simulink model "accumulator_thermal_model"  (R2022b)
settings: Solver=VariableStepAuto  StartTime=0.0  StopTime=Tend  RelTol=1e-7  AbsTol=1e-7
InitFcn:
  | HT06_Simulink_Setup
values from neighbouring files (symbols this model uses):
  AH = 18    [HT06_Simulink_Setup.m]
  convectionArea = baseplateArea/126    (= 0.00235277777778)    [Copy_of_Simulink_Setup.m]    (also in HT06_Simulink_Setup.m = 0.00297619047619; Simulink_Setup.m = 0.00297619047619)
  SOC0 = 1    [HT06_Simulink_Setup.m]
  startTempC = 23.5    [Copy_of_Simulink_Setup.m]    (also in HT06_Simulink_Setup.m = 23.3; Simulink_Setup.m)
  tabResis = 0.00009    (= 9e-05)    [Copy_of_Simulink_Setup.m]    (also in HT06_Simulink_Setup.m = 0.0001; Simulink_Setup.m)
undefined symbols (not defined in the file or in its folder): DiscIntNeverNeededParam, S
libraries: fl_lib x49, nesl_utility x18, ee_lib x2
settings Model: Creator=elrii  LastModifiedBy=dknight34
settings SolverCC: AutoScaleAbsTol=off  AlgebraicLoopSolver=TrustRegion
settings DataIOCC: ReturnWorkspaceOutputsName=tp141c3138_a421_409b_bff7_0e00beb78378
settings DebuggingCC: UnconnectedInputMsg=warning  UnconnectedOutputMsg=warning  UnconnectedLineMsg=warning  SymbolicDimsDataTypeCodeGenerationDiagnostic=none  SFMachineParentedDataDiag=warning
settings ModelReferenceCC: EnableRefExpFcnMdlSchedulingChecks=on
settings SFSimCC: CustomCodeUndefinedFunction=UseInterfaceOnly
settings RTWCC: DLArmComputeVersion=19.05
settings SimscapeCC: SimscapeLogType=all  SimscapeLogSimulationStatistics=on  SimscapeLogDataHistory=10000

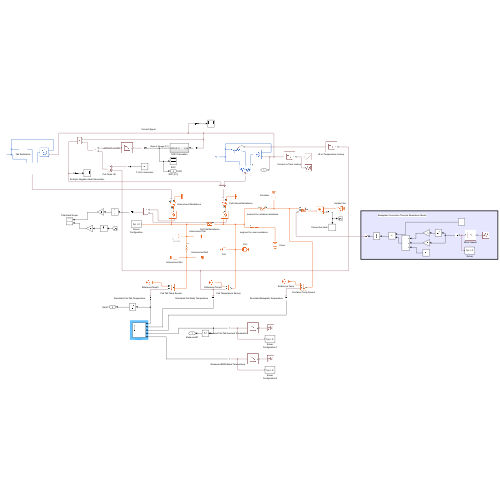
[thumbnail: Simulink's stored preview of the top-level diagram]
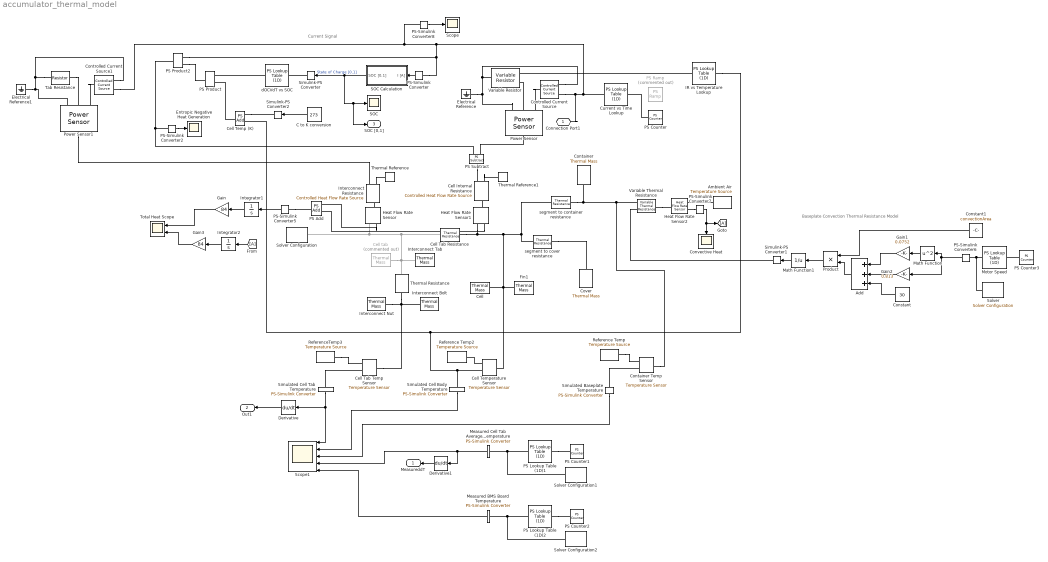
== system accumulator_thermal_model ==
  note: Baseplate Convection Thermal Resistance Model
  note: Current Signal
  " Fin1" : fl_lib/Thermal/Thermal Elements/Thermal Mass  mass=mFin kg  sp_heat=cAl J/kg/K  num_ports=foundation.enum.numPorts2.one  T_specify=on  T_priority=High  T=startTempC degC  T_nominal_specify=off  T_nominal_unit=K  T_nominal_value=1  Q_specify=off  Q_priority=None  Q=0 W  Q_nominal_specify=off  Q_nominal_unit=W  Q_nominal_value=1
  Add : Sum  Inputs=+++
  Ambient Air : fl_lib/Thermal/Thermal Sources/Temperature Source  temperature=startTempC degC
  C to K conversion : Constant  Value=273
  "Cell " : fl_lib/Thermal/Thermal Elements/Thermal Mass  mass=mCell kg  sp_heat=cCell J/kg/K  num_ports=foundation.enum.numPorts2.one  T_specify=on  T_priority=High  T=startTempC degC  T_nominal_specify=off  T_nominal_unit=K  T_nominal_value=1  Q_specify=off  Q_priority=None  Q=0 W  Q_nominal_specify=off  Q_nominal_unit=W  Q_nominal_value=1
  Cell Internal Resistance : fl_lib/Thermal/Thermal Sources/Controlled Heat Flow Rate Source
  Cell Tab Resistance : fl_lib/Thermal/Thermal Elements/Thermal Resistance  resistance=R_tc K/W  T_specify=off  T_priority=None  T=0 K  T_nominal_specify=off  T_nominal_unit=K  T_nominal_value=1  Q_specify=off  Q_priority=None  Q=0 W  Q_nominal_specify=off  Q_nominal_unit=W  Q_nominal_value=1
  Cell Tab Temp Sensor : fl_lib/Thermal/Thermal Sensors/Temperature Sensor
  Cell Temp (K) : fl_lib/Physical Signals/Functions/PS Add
  Cell Temperature Sensor : fl_lib/Thermal/Thermal Sensors/Temperature Sensor
  Cell tab : fl_lib/Thermal/Thermal Elements/Thermal Mass  Commented=on  mass=cellTabThermalMass kg  sp_heat=cCu J/kg/K  num_ports=foundation.enum.numPorts2.one  T_specify=on  T_priority=High  T=startTempC degC  T_nominal_specify=off  T_nominal_unit=K  T_nominal_value=1  Q_specify=off  Q_priority=None  Q=0 W  Q_nominal_specify=off  Q_nominal_unit=W  Q_nominal_value=1
  Constant : Constant  Value=30
  Constant1 : Constant  Value=convectionArea
  Container : fl_lib/Thermal/Thermal Elements/Thermal Mass  mass=mContainerAdj kg  sp_heat=cAl J/kg/K  num_ports=foundation.enum.numPorts2.one  T_specify=on  T_priority=High  T=startTempC degC  T_nominal_specify=off  T_nominal_unit=K  T_nominal_value=1  Q_specify=off  Q_priority=None  Q=0 W  Q_nominal_specify=off  Q_nominal_unit=W  Q_nominal_value=1
  Container Temp Sensor : fl_lib/Thermal/Thermal Sensors/Temperature Sensor
  Controlled Current Source : fl_lib/Electrical/Electrical Sources/Controlled Current Source
  Controlled Current Source1 : fl_lib/Electrical/Electrical Sources/Controlled Current Source
  Convective Heat : Scope
  Cover : fl_lib/Thermal/Thermal Elements/Thermal Mass  mass=mCoverAdj kg  sp_heat=cAl J/kg/K  num_ports=foundation.enum.numPorts2.one  T_specify=on  T_priority=High  T=startTempC degC  T_nominal_specify=off  T_nominal_unit=K  T_nominal_value=1  Q_specify=off  Q_priority=None  Q=0 W  Q_nominal_specify=off  Q_nominal_unit=W  Q_nominal_value=1
  Current vs Time Lookup : fl_lib/Physical Signals/Lookup Tables/PS Lookup Table (1D)  x=emTime  f=emCurrent A  interp_method=simscape.enum.interpolation.linear  extrap_method=simscape.enum.extrapolation.nearest
  Derivative : Derivative
  Derivative1 : Derivative
  Electrical Reference : fl_lib/Electrical/Electrical Elements/Electrical Reference
  Electrical Reference1 : fl_lib/Electrical/Electrical Elements/Electrical Reference
  Entropic Negative Heat Generation : Scope
  From : From
  Gain : Gain  Gain=84
  Gain1 : Gain  Gain=0.0752
  Gain2 : Gain  Gain=0.813
  Gain3 : Gain  Gain=84
  Goto : Goto
  Heat Flow Rate Sensor : fl_lib/Thermal/Thermal Sensors/Heat Flow Rate Sensor
  Heat Flow Rate Sensor1 : fl_lib/Thermal/Thermal Sensors/Heat Flow Rate Sensor
  Heat Flow Rate Sensor2 : fl_lib/Thermal/Thermal Sensors/Heat Flow Rate Sensor
  IR vs Temperature Lookup : fl_lib/Physical Signals/Lookup Tables/PS Lookup Table (1D)  x=tempVec K  f=IRVec Ohm  interp_method=simscape.enum.interpolation.linear  extrap_method=simscape.enum.extrapolation.nearest
  Integrator1 : Integrator
  Integrator2 : Integrator
  Interconnect Bolt : fl_lib/Thermal/Thermal Elements/Thermal Mass  mass=mInterconnectBoltTotal kg  sp_heat=cSt J/kg/K  num_ports=foundation.enum.numPorts2.one  T_specify=on  T_priority=High  T=startTempC degC  T_nominal_specify=off  T_nominal_unit=K  T_nominal_value=1  Q_specify=off  Q_priority=None  Q=0 W  Q_nominal_specify=off  Q_nominal_unit=W  Q_nominal_value=1
  Interconnect Nut : fl_lib/Thermal/Thermal Elements/Thermal Mass  mass=mInterconnectNutTotal kg  sp_heat=cSt J/kg/K  num_ports=foundation.enum.numPorts2.one  T_specify=on  T_priority=High  T=startTempC degC  T_nominal_specify=off  T_nominal_unit=K  T_nominal_value=1  Q_specify=off  Q_priority=None  Q=0 W  Q_nominal_specify=off  Q_nominal_unit=W  Q_nominal_value=1
  Interconnect Resistance : fl_lib/Thermal/Thermal Sources/Controlled Heat Flow Rate Source
  Interconnect Tab : fl_lib/Thermal/Thermal Elements/Thermal Mass  mass=mInterconnect kg  sp_heat=cAl J/kg/K  num_ports=foundation.enum.numPorts2.one  T_specify=on  T_priority=High  T=startTempC degC  T_nominal_specify=off  T_nominal_unit=K  T_nominal_value=1  Q_specify=off  Q_priority=None  Q=0 W  Q_nominal_specify=off  Q_nominal_unit=W  Q_nominal_value=1
  Math Function : Math  Operator=square
  Math Function1 : Math  Operator=reciprocal
  Measured BMS Board Temperature : nesl_utility/PS-Simulink Converter  PhysicalDomain=network_engine_domain  SubClassName=ps_output  LeftPortType=input  RightPortType=output  PseudoPeriodic=off  Frequencies=[]  VectorFormat=1-D array  Unit=inherit  AffineConversion=off
  Measured Cell Tab Average Temperature : nesl_utility/PS-Simulink Converter  PhysicalDomain=network_engine_domain  SubClassName=ps_output  LeftPortType=input  RightPortType=output  PseudoPeriodic=off  Frequencies=[]  VectorFormat=1-D array  Unit=inherit  AffineConversion=off
  Motor Speed : fl_lib/Physical Signals/Lookup Tables/PS Lookup Table (1D)  x=S.vehicle_speed(:,1)  f=S.vehicle_speed(:,2)  interp_method=simscape.enum.interpolation.linear  extrap_method=simscape.enum.extrapolation.nearest
  PS Add : fl_lib/Physical Signals/Functions/PS Add
  PS Counter : fl_lib/Physical Signals/Sources/PS Counter  sample_time=1 s  init_val=0  reset_val=0  max_val=intmax
      settings: InternalSimscapePortConfiguration="{\"Bottom\":[],\"Left\":[],\"Right\":[{\"id\":\"Y\",\"label\":\"Y\",\"type\":\"output\"}],\"Top\":[]}"
  PS Counter1 : fl_lib/Physical Signals/Sources/PS Counter  sample_time=1 s  init_val=1  reset_val=0  max_val=100000
      settings: InternalSimscapePortConfiguration="{\"Bottom\":[],\"Left\":[],\"Right\":[{\"id\":\"Y\",\"label\":\"Y\",\"type\":\"output\"}],\"Top\":[]}"
  PS Counter2 : fl_lib/Physical Signals/Sources/PS Counter  sample_time=1 s  init_val=1  reset_val=0  max_val=100000
      settings: InternalSimscapePortConfiguration="{\"Bottom\":[],\"Left\":[],\"Right\":[{\"id\":\"Y\",\"label\":\"Y\",\"type\":\"output\"}],\"Top\":[]}"
  PS Counter3 : fl_lib/Physical Signals/Sources/PS Counter  sample_time=1 s  init_val=0  reset_val=0  max_val=intmax
      settings: InternalSimscapePortConfiguration="{\"Bottom\":[],\"Left\":[],\"Right\":[{\"id\":\"Y\",\"label\":\"Y\",\"type\":\"output\"}],\"Top\":[]}"
  PS Lookup Table (1D)1 : fl_lib/Physical Signals/Lookup Tables/PS Lookup Table (1D)  x=time  f=tempInterp  interp_method=simscape.enum.interpolation.linear  extrap_method=simscape.enum.extrapolation.nearest
  PS Lookup Table (1D)2 : fl_lib/Physical Signals/Lookup Tables/PS Lookup Table (1D)  x=time  f=accAirTempInterp  interp_method=simscape.enum.interpolation.linear  extrap_method=simscape.enum.extrapolation.nearest
  PS Product : fl_lib/Physical Signals/Functions/PS Product
  PS Product2 : fl_lib/Physical Signals/Functions/PS Product
  PS Ramp : fl_lib/Physical Signals/Sources/PS Ramp  Commented=on  slope=1 1/s  start_time=0 s  initial_output=0
  PS Subtract : fl_lib/Physical Signals/Functions/PS Subtract
  PS-Simulink Converter : nesl_utility/PS-Simulink Converter  PhysicalDomain=network_engine_domain  SubClassName=ps_output  LeftPortType=input  RightPortType=output  PseudoPeriodic=off  Frequencies=[]  VectorFormat=1-D array  Unit=inherit  AffineConversion=off
  PS-Simulink Converter2 : nesl_utility/PS-Simulink Converter  PhysicalDomain=network_engine_domain  SubClassName=ps_output  LeftPortType=input  RightPortType=output  PseudoPeriodic=off  Frequencies=[]  VectorFormat=1-D array  Unit=inherit  AffineConversion=off
  PS-Simulink Converter5 : nesl_utility/PS-Simulink Converter  PhysicalDomain=network_engine_domain  SubClassName=ps_output  LeftPortType=input  RightPortType=output  PseudoPeriodic=off  Frequencies=[]  VectorFormat=1-D array  Unit=inherit  AffineConversion=off
  PS-Simulink Converter6 : nesl_utility/PS-Simulink Converter  PhysicalDomain=network_engine_domain  SubClassName=ps_output  LeftPortType=input  RightPortType=output  PseudoPeriodic=off  Frequencies=[]  VectorFormat=inherit  Unit=inherit  AffineConversion=off
  PS-Simulink Converter7 : nesl_utility/PS-Simulink Converter  PhysicalDomain=network_engine_domain  SubClassName=ps_output  LeftPortType=input  RightPortType=output  PseudoPeriodic=off  Frequencies=[]  VectorFormat=inherit  Unit=inherit  AffineConversion=off
  PS-Simulink Converter8 : nesl_utility/PS-Simulink Converter  PhysicalDomain=network_engine_domain  SubClassName=ps_output  LeftPortType=input  RightPortType=output  PseudoPeriodic=off  Frequencies=[]  VectorFormat=inherit  Unit=inherit  AffineConversion=off
  Power Sensor : ee_lib/Sensors & Transducers/Power Sensor  measurement_type=1  averaging_period=1e-4 s
  Power Sensor1 : ee_lib/Sensors & Transducers/Power Sensor  measurement_type=1  averaging_period=1e-4 s
  Product : Product
  Reference Temp : fl_lib/Thermal/Thermal Sources/Temperature Source  temperature=0 degC
  Reference Temp2 : fl_lib/Thermal/Thermal Sources/Temperature Source  temperature=0 degC
  ReferenceTemp3 : fl_lib/Thermal/Thermal Sources/Temperature Source  temperature=0 degC
  SOC : Scope
  SOC Calculation : Subsystem
  Scope : Scope
  Scope1 : Scope  NumInputPorts=5
  Simulated Baseplate Temperature : nesl_utility/PS-Simulink Converter  PhysicalDomain=network_engine_domain  SubClassName=ps_output  LeftPortType=input  RightPortType=output  PseudoPeriodic=off  Frequencies=[]  VectorFormat=1-D array  Unit=inherit  AffineConversion=off
  Simulated Cell Body Temperature : nesl_utility/PS-Simulink Converter  PhysicalDomain=network_engine_domain  SubClassName=ps_output  LeftPortType=input  RightPortType=output  PseudoPeriodic=off  Frequencies=[]  VectorFormat=1-D array  Unit=inherit  AffineConversion=off
  Simulated Cell Tab Temperature : nesl_utility/PS-Simulink Converter  PhysicalDomain=network_engine_domain  SubClassName=ps_output  LeftPortType=input  RightPortType=output  PseudoPeriodic=off  Frequencies=[]  VectorFormat=1-D array  Unit=inherit  AffineConversion=off
  Simulink-PS Converter : nesl_utility/Simulink-PS Converter  PhysicalDomain=network_engine_domain  SubClassName=ps_input  LeftPortType=input  RightPortType=output  PseudoPeriodic=off  Frequencies=[]  NoiseDistribution=none  NoiseParameters=[]  Unit=1  AffineConversion=off  FilteringAndDerivatives=provide  SimscapeFilterOrder=1  InputFilterTimeConstant=0.001  UdotUserProvided=0
  Simulink-PS Converter1 : nesl_utility/Simulink-PS Converter  PhysicalDomain=network_engine_domain  SubClassName=ps_input  LeftPortType=input  RightPortType=output  PseudoPeriodic=off  Frequencies=[]  NoiseDistribution=none  NoiseParameters=[]  Unit=K/W  AffineConversion=off  FilteringAndDerivatives=provide  SimscapeFilterOrder=1  InputFilterTimeConstant=0.001  UdotUserProvided=0
  Simulink-PS Converter2 : nesl_utility/Simulink-PS Converter  PhysicalDomain=network_engine_domain  SubClassName=ps_input  LeftPortType=input  RightPortType=output  PseudoPeriodic=off  Frequencies=[]  NoiseDistribution=none  NoiseParameters=[]  Unit=K  AffineConversion=off  FilteringAndDerivatives=provide  SimscapeFilterOrder=1  InputFilterTimeConstant=0.001  UdotUserProvided=0
  Solver : nesl_utility/Solver Configuration  PhysicalDomain=network_engine_domain  SubClassName=solver  LeftPortType=input  RightPortType=generic  Tones=[]  Harmonics=[]  SimulateNoise=off  Profile=off  UseLocalSampling=off  EnableSwitchedLinearOptims=on  FrequencyDomain=off  UseCCode=off  RelTol=0.001  AbsTol=1e-06  MinStep=1e-09  ToWorkspace=off  RevertToSquareIcSolve=off  NumHomotopyIterations=100  PhasorMode=off  PhasorModeNumHarmonics=1  ConsistencySolver=NEWTON_FTOL  IndexReductionMethod=DerivativeReplacement  DoDC=off  ResidualTolerance=1e-09  ConsistencyTolSource=GLOBAL  ConsistencyAbsTol=0.001  ConsistencyRelTol=0.001  ConsistencyTolFactor=0.001  UseLocalSolver=off  LocalSolverChoice=NE_BACKWARD_EULER_ADVANCER  ResolveIndetEquations=on  FunctionEvalNumThread=1  LocalSolverSampleTime=0.001  DoFixedCost=off  MaxNonlinIter=3  MaxModeIter=2  ComputeImpulses=off  ImpulseIterations=2  LinearAlgebra=auto  LinearAlgebraNumThread=0  EquationFormulation=NE_TIME_EF  DelaysMemoryBudget=1024  AutomaticFiltering=on  FilteringTimeConstant=0.001  PartitionStorageMethod=AS_NEEDED  PartitionMemoryBudget=1024  PartitionMethod=ROBUST
  Solver Configuration : nesl_utility/Solver Configuration  PhysicalDomain=network_engine_domain  SubClassName=solver  LeftPortType=input  RightPortType=generic  Tones=[]  Harmonics=[]  SimulateNoise=off  Profile=off  UseLocalSampling=off  EnableSwitchedLinearOptims=on  FrequencyDomain=off  UseCCode=off  RelTol=0.001  AbsTol=1e-06  MinStep=1e-09  ToWorkspace=off  RevertToSquareIcSolve=off  NumHomotopyIterations=100  PhasorMode=off  PhasorModeNumHarmonics=1  ConsistencySolver=NEWTON_FTOL  IndexReductionMethod=DerivativeReplacement  DoDC=off  ResidualTolerance=1e-012  ConsistencyTolSource=GLOBAL  ConsistencyAbsTol=0.001  ConsistencyRelTol=0.001  ConsistencyTolFactor=0.001  UseLocalSolver=off  LocalSolverChoice=NE_BACKWARD_EULER_ADVANCER  ResolveIndetEquations=on  FunctionEvalNumThread=1  LocalSolverSampleTime=0.001  DoFixedCost=off  MaxNonlinIter=3  MaxModeIter=2  ComputeImpulses=off  ImpulseIterations=2  LinearAlgebra=auto  LinearAlgebraNumThread=0  EquationFormulation=NE_TIME_EF  DelaysMemoryBudget=1024  AutomaticFiltering=on  FilteringTimeConstant=0.001  PartitionStorageMethod=AS_NEEDED  PartitionMemoryBudget=1024  PartitionMethod=ROBUST
  Solver Configuration1 : nesl_utility/Solver Configuration  PhysicalDomain=network_engine_domain  SubClassName=solver  LeftPortType=input  RightPortType=generic  Tones=[]  Harmonics=[]  SimulateNoise=off  Profile=off  UseLocalSampling=off  EnableSwitchedLinearOptims=on  FrequencyDomain=off  UseCCode=off  RelTol=0.001  AbsTol=1e-06  MinStep=1e-09  ToWorkspace=off  RevertToSquareIcSolve=off  NumHomotopyIterations=100  PhasorMode=off  PhasorModeNumHarmonics=1  ConsistencySolver=NEWTON_FTOL  IndexReductionMethod=DerivativeReplacement  DoDC=off  ResidualTolerance=1e-09  ConsistencyTolSource=GLOBAL  ConsistencyAbsTol=0.001  ConsistencyRelTol=0.001  ConsistencyTolFactor=0.001  UseLocalSolver=off  LocalSolverChoice=NE_BACKWARD_EULER_ADVANCER  ResolveIndetEquations=on  FunctionEvalNumThread=1  LocalSolverSampleTime=0.001  DoFixedCost=off  MaxNonlinIter=3  MaxModeIter=2  ComputeImpulses=off  ImpulseIterations=2  LinearAlgebra=auto  LinearAlgebraNumThread=0  EquationFormulation=NE_TIME_EF  DelaysMemoryBudget=1024  AutomaticFiltering=on  FilteringTimeConstant=0.001  PartitionStorageMethod=AS_NEEDED  PartitionMemoryBudget=1024  PartitionMethod=ROBUST
  Solver Configuration2 : nesl_utility/Solver Configuration  PhysicalDomain=network_engine_domain  SubClassName=solver  LeftPortType=input  RightPortType=generic  Tones=[]  Harmonics=[]  SimulateNoise=off  Profile=off  UseLocalSampling=off  EnableSwitchedLinearOptims=on  FrequencyDomain=off  UseCCode=off  RelTol=0.001  AbsTol=1e-06  MinStep=1e-09  ToWorkspace=off  RevertToSquareIcSolve=off  NumHomotopyIterations=100  PhasorMode=off  PhasorModeNumHarmonics=1  ConsistencySolver=NEWTON_FTOL  IndexReductionMethod=DerivativeReplacement  DoDC=off  ResidualTolerance=1e-09  ConsistencyTolSource=GLOBAL  ConsistencyAbsTol=0.001  ConsistencyRelTol=0.001  ConsistencyTolFactor=0.001  UseLocalSolver=off  LocalSolverChoice=NE_BACKWARD_EULER_ADVANCER  ResolveIndetEquations=on  FunctionEvalNumThread=1  LocalSolverSampleTime=0.001  DoFixedCost=off  MaxNonlinIter=3  MaxModeIter=2  ComputeImpulses=off  ImpulseIterations=2  LinearAlgebra=auto  LinearAlgebraNumThread=0  EquationFormulation=NE_TIME_EF  DelaysMemoryBudget=1024  AutomaticFiltering=on  FilteringTimeConstant=0.001  PartitionStorageMethod=AS_NEEDED  PartitionMemoryBudget=1024  PartitionMethod=ROBUST
  Tab Resistance : fl_lib/Electrical/Electrical Elements/Resistor  R=tabResis Ohm  i_specify=off  i_priority=None  i=0 A  i_nominal_specify=off  i_nominal_unit=A  i_nominal_value=1  v_specify=off  v_priority=None  v=0 V  v_nominal_specify=off  v_nominal_unit=V  v_nominal_value=1  mask(Resistor){}
  Thermal Reference : fl_lib/Thermal/Thermal Elements/Thermal Reference
  Thermal Reference1 : fl_lib/Thermal/Thermal Elements/Thermal Reference
  Thermal Resistance : fl_lib/Thermal/Thermal Elements/Thermal Resistance  resistance=thermistorContactRes K/W  T_specify=off  T_priority=None  T=0 K  T_nominal_specify=off  T_nominal_unit=K  T_nominal_value=1  Q_specify=off  Q_priority=None  Q=0 W  Q_nominal_specify=off  Q_nominal_unit=W  Q_nominal_value=1
  Total Heat Scope : Scope  NumInputPorts=2
  Variable Resistor : fl_lib/Electrical/Electrical Elements/Variable Resistor  Rmin=0 Ohm  i_specify=off  i_priority=None  i=0 A  i_nominal_specify=off  i_nominal_unit=A  i_nominal_value=1  v_specify=off  v_priority=None  v=0 V  v_nominal_specify=off  v_nominal_unit=V  v_nominal_value=1
  Variable Thermal Resistance : fl_lib/Thermal/Thermal Elements/Variable Thermal Resistance  R_min=0 K/W  T_specify=off  T_priority=None  T=0 K  T_nominal_specify=off  T_nominal_unit=K  T_nominal_value=1  Q_specify=off  Q_priority=None  Q=0 W  Q_nominal_specify=off  Q_nominal_unit=W  Q_nominal_value=1
      settings: InternalSimscapePortConfiguration="{\"Bottom\":[],\"Left\":[{\"id\":\"A\",\"label\":\"A\",\"type\":\"foundation.thermal.thermal\"},{\"id\":\"R\",\"label\":\"R\",\"type\":\"input\"}],\"Right\":[{\"id\":\"B\",\"label\":\"B\",\"type\":\"foundation.thermal.thermal\"}],\"Top\":[]}"
  dOCVdT vs SOC : fl_lib/Physical Signals/Lookup Tables/PS Lookup Table (1D)  x=SOC  f=dOCVdT V/K  interp_method=simscape.enum.interpolation.linear  extrap_method=simscape.enum.extrapolation.linear
  segment to container resistance : fl_lib/Thermal/Thermal Elements/Thermal Resistance  resistance=R_cb K/W  T_specify=off  T_priority=None  T=0 K  T_nominal_specify=off  T_nominal_unit=K  T_nominal_value=1  Q_specify=off  Q_priority=None  Q=0 W  Q_nominal_specify=off  Q_nominal_unit=W  Q_nominal_value=1
  segment to cover resistance : fl_lib/Thermal/Thermal Elements/Thermal Resistance  resistance=R_cb K/W  T_specify=off  T_priority=None  T=0 K  T_nominal_specify=off  T_nominal_unit=K  T_nominal_value=1  Q_specify=off  Q_priority=None  Q=0 W  Q_nominal_specify=off  Q_nominal_unit=W  Q_nominal_value=1
  Connection Port1 : PMIOPort  Side=Left
  MeasureddT : Outport
  Out1 : Outport  Port=2  SignalName=SimdT
  SOC [0,1] : Outport  Port=3  SignalName=SOC
  wires:
  Simulated Cell Tab Temperature/1 -> Scope1/1, Derivative/1
  Measured Cell Tab Average Temperature/1 -> Scope1/4, Derivative1/1
  PS-Simulink Converter/1 -> SOC Calculation/1(I [A])
  SOC Calculation/1(SOC [0,1]) -> Simulink-PS Converter/1, SOC [0,1]/1, SOC/1  "State of Charge [0,1]"
  C to K conversion/1 -> Simulink-PS Converter2/1
  PS-Simulink Converter2/1 -> Entropic Negative Heat Generation/1
  Simulated Cell Body Temperature/1 -> Scope1/2
  PS-Simulink Converter5/1 -> Integrator1/1
  Integrator1/1 -> Gain/1
  Gain/1 -> Total Heat Scope/1
  Simulated Baseplate Temperature/1 -> Scope1/3
  Measured BMS Board Temperature/1 -> Scope1/5
  PS-Simulink Converter6/1 -> Gain2/1, Math Function/1
  Math Function/1 -> Gain1/1
  Gain1/1 -> Add/1
  Gain2/1 -> Add/2
  Constant/1 -> Add/3
  Constant1/1 -> Product/1
  Add/1 -> Product/2
  Product/1 -> Math Function1/1
  Math Function1/1 -> Simulink-PS Converter1/1
  PS-Simulink Converter7/1 -> Goto/1, Convective Heat/1
  From/1 -> Integrator2/1
  Integrator2/1 -> Gain3/1
  Gain3/1 -> Total Heat Scope/2
  Derivative/1 -> Out1/1
  Derivative1/1 -> MeasureddT/1
  PS-Simulink Converter8/1 -> Scope/1
  connections:
  segment to cover resistance/LConn1 -- segment to container resistance/LConn1 -- Heat Flow Rate Sensor1/RConn2 -- Cell Tab Resistance/RConn1 -- Cell Temperature Sensor/LConn1 -- " Fin1"/LConn1 -- "Cell "/LConn1
  Cell tab/LConn1 -- Thermal Resistance/LConn1 -- Interconnect Tab/LConn1 -- Heat Flow Rate Sensor/RConn2 -- Solver Configuration/RConn1 -- Cell Tab Resistance/LConn1
  Controlled Current Source/LConn1 -- Power Sensor/LConn1
  Power Sensor/LConn2 -- Variable Resistor/LConn2
  Power Sensor/LConn3 -- Electrical Reference/LConn1 -- Controlled Current Source/RConn2 -- Variable Resistor/RConn1
  Tab Resistance/RConn1 -- Controlled Current Source1/RConn2 -- Power Sensor1/LConn3 -- Electrical Reference1/LConn1
  Tab Resistance/LConn1 -- Power Sensor1/LConn2
  Controlled Current Source1/LConn1 -- Power Sensor1/LConn1
  Power Sensor1/RConn1 -- Interconnect Resistance/RConn1
  Interconnect Resistance/RConn2 -- Thermal Reference/LConn1
  segment to container resistance/RConn1 -- Container Temp Sensor/LConn1 -- Variable Thermal Resistance/LConn1 -- Container/LConn1
  Controlled Current Source/RConn1 -- Connection Port1/RConn1 -- Current vs Time Lookup/RConn1 -- PS-Simulink Converter8/LConn1 -- Controlled Current Source1/RConn1 -- PS-Simulink Converter/LConn1 -- PS Product2/LConn1
  ReferenceTemp3/LConn1 -- Cell Tab Temp Sensor/RConn1
  PS Lookup Table (1D)1/RConn1 -- Solver Configuration1/RConn1 -- Measured Cell Tab Average Temperature/LConn1
  PS Lookup Table (1D)1/LConn1 -- PS Counter1/RConn1
  Simulated Cell Tab Temperature/LConn1 -- Cell Tab Temp Sensor/RConn2
  Simulink-PS Converter/RConn1 -- dOCVdT vs SOC/LConn1
  dOCVdT vs SOC/RConn1 -- PS Product/LConn1
  PS Product2/LConn2 -- PS Product/RConn1
  PS Subtract/LConn1 -- Power Sensor/RConn1
  PS Subtract/RConn1 -- Cell Internal Resistance/RConn1
  Cell Temp (K)/LConn1 -- Simulink-PS Converter2/RConn1
  Cell Temp (K)/RConn1 -- PS Product/LConn2
  Simulated Baseplate Temperature/LConn1 -- Container Temp Sensor/RConn2
  PS Subtract/LConn2 -- PS Product2/RConn1 -- PS-Simulink Converter2/LConn1
  IR vs Temperature Lookup/RConn1 -- Variable Resistor/LConn1
  Cell Temperature Sensor/RConn2 -- Simulated Cell Body Temperature/LConn1 -- IR vs Temperature Lookup/LConn1 -- Cell Temp (K)/LConn2
  segment to cover resistance/RConn1 -- Cover/LConn1
  Interconnect Nut/LConn1 -- Cell Tab Temp Sensor/LConn1 -- Thermal Resistance/RConn1 -- Interconnect Bolt/LConn1
  Reference Temp/LConn1 -- Container Temp Sensor/RConn1
  Cell Temperature Sensor/RConn1 -- Reference Temp2/LConn1
  Cell Internal Resistance/RConn2 -- Thermal Reference1/LConn1
  Interconnect Resistance/LConn1 -- Heat Flow Rate Sensor/LConn1
  Cell Internal Resistance/LConn1 -- Heat Flow Rate Sensor1/LConn1
  Heat Flow Rate Sensor1/RConn1 -- PS Add/LConn1
  Heat Flow Rate Sensor/RConn1 -- PS Add/LConn2
  PS-Simulink Converter5/LConn1 -- PS Add/RConn1
  Measured BMS Board Temperature/LConn1 -- PS Lookup Table (1D)2/RConn1 -- Solver Configuration2/RConn1
  PS Lookup Table (1D)2/LConn1 -- PS Counter2/RConn1
  PS Counter3/RConn1 -- Motor Speed/LConn1
  PS-Simulink Converter6/LConn1 -- Solver/RConn1 -- Motor Speed/RConn1
  Simulink-PS Converter1/RConn1 -- Variable Thermal Resistance/LConn2
  Variable Thermal Resistance/RConn1 -- Heat Flow Rate Sensor2/LConn1
  Heat Flow Rate Sensor2/RConn2 -- Ambient Air/LConn1
  Heat Flow Rate Sensor2/RConn1 -- PS-Simulink Converter7/LConn1
  PS Counter/RConn1 -- Current vs Time Lookup/LConn1

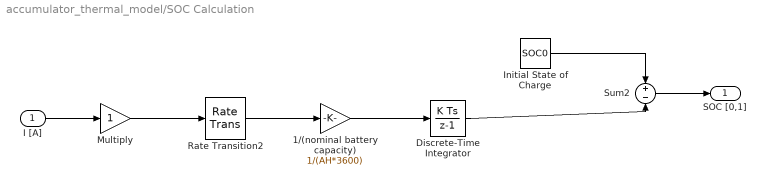
== system accumulator_thermal_model/SOC Calculation ==
  I [A] : Inport
  1/(nominal battery capacity) : Gain  Gain=1/(AH*3600)
  Discrete-Time Integrator : DiscreteIntegrator  SampleTime=-1  ICPrevOutput=DiscIntNeverNeededParam  ICPrevScaledInput=DiscIntNeverNeededParam
  Initial State of Charge : Constant  Value=SOC0
  Multiply : Gain
  Rate Transition2 : RateTransition
  Sum2 : Sum  Inputs=+-
  SOC [0,1] : Outport  VectorParamsAs1DForOutWhenUnconnected=off
  wires:
  Rate Transition2/1 -> 1/(nominal battery capacity)/1
  1/(nominal battery capacity)/1 -> Discrete-Time Integrator/1
  Initial State of Charge/1 -> Sum2/1
  Discrete-Time Integrator/1 -> Sum2/2
  Sum2/1 -> SOC [0,1]/1
  I [A]/1 -> Multiply/1
  Multiply/1 -> Rate Transition2/1
